simulink model "analog_ext2"  (Simulink 7.6)
settings: Solver=FixedStepDiscrete  StartTime=0.0  StopTime=10000  FixedStep=1  RelTol=1e-3
libraries: simulink x8
settings Model: Creator=jordan  LastModifiedBy=jordan
settings DataIOCC: LimitDataPoints=off  SaveOutput=off  SignalLogging=off  DSMLogging=off  SaveTime=off
settings OptimizationCC: BlockReduction=off  ConditionallyExecuteInputs=off

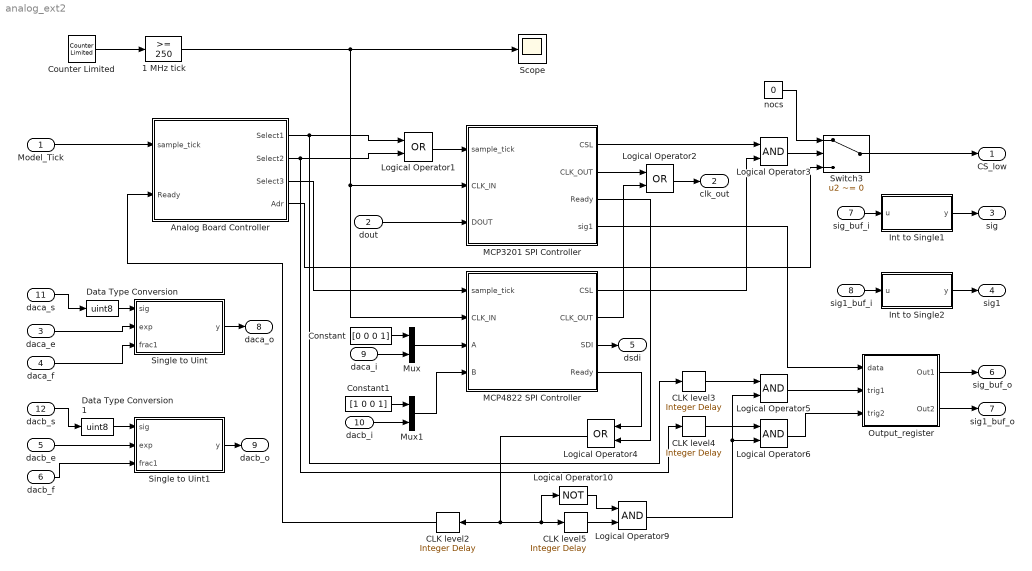
== system analog_ext2 ==
  Model_Tick : Inport  OutDataTypeStr=boolean
  dout : Inport  Port=2  OutDataTypeStr=boolean
  daca_e : Inport  Port=3  OutDataTypeStr=uint8
  daca_f : Inport  Port=4  OutDataTypeStr=fixdt(0,24,0)
  dacb_e : Inport  Port=5  OutDataTypeStr=uint8
  dacb_f : Inport  Port=6  OutDataTypeStr=fixdt(0,24,0)
  sig_buf_i : Inport  Port=7  OutDataTypeStr=fixdt(0,12,0)
  sig1_buf_i : Inport  Port=8  OutDataTypeStr=fixdt(0,12,0)
  daca_i : Inport  Port=9  OutDataTypeStr=boolean  PortDimensions=12
  dacb_i : Inport  Port=10  OutDataTypeStr=boolean  PortDimensions=12
  daca_s : Inport  Port=11  OutDataTypeStr=boolean
  dacb_s : Inport  Port=12  OutDataTypeStr=boolean
  1 MHz tick : simulink/Logic and Bit Operations/Compare To Constant  SystemSampleTime=-1  relop=>=  const=250  LogicOutDataTypeMode=boolean
  Analog Board Controller : Stateflow chart  TreatAsAtomicUnit=on
  CLK level{2..5} (4 alike) : simulink/Discrete/Integer Delay  NumDelays=1  vinit=0.0  samptime=-1
  Constant : Constant  Value=[0 0 0 1]  OutDataTypeStr=boolean
  Constant1 : Constant  Value=[1 0 0 1]  OutDataTypeStr=boolean
  Counter Limited : simulink/Sources/Counter Limited  SystemSampleTime=-1  uplimit=500  tsamp=-1
  Data Type Conversion : DataTypeConversion  OutDataTypeStr=uint8
  Data Type Conversion1 : DataTypeConversion  OutDataTypeStr=uint8
  Int to Single1 : Stateflow chart  TreatAsAtomicUnit=on
  Int to Single2 : Stateflow chart  TreatAsAtomicUnit=on
  Logical Operator1 : Logic  Operator=OR  AllPortsSameDT=off  OutDataTypeStr=boolean
  Logical Operator10 : Logic  Operator=NOT  AllPortsSameDT=off  OutDataTypeStr=boolean
  Logical Operator2 : Logic  Operator=OR  AllPortsSameDT=off  OutDataTypeStr=boolean
  Logical Operator{3,5..6,9} (4 alike) : Logic  AllPortsSameDT=off  OutDataTypeStr=boolean
  Logical Operator4 : Logic  Operator=OR  AllPortsSameDT=off  OutDataTypeStr=boolean
  MCP3201 SPI Controller : Stateflow chart  TreatAsAtomicUnit=on
  MCP4822 SPI Controller : Stateflow chart  TreatAsAtomicUnit=on
  Mux : Mux  Inputs=2
  Mux1 : Mux  Inputs=2
  Output_register : Subsystem
  Scope : Scope
  Single to Uint : Stateflow chart  TreatAsAtomicUnit=on
  Single to Uint1 : Stateflow chart  TreatAsAtomicUnit=on
  Switch3 : Switch  Criteria=u2 ~= 0
  nocs : Constant  Value=0  OutDataTypeStr=fixdt(0,3,0)
  CS_low : Outport  OutDataTypeStr=fixdt(0,3,0)
  clk_out : Outport  Port=2  OutDataTypeStr=boolean
  sig : Outport  Port=3  OutDataTypeStr=uint32  PortDimensions=1
  sig1 : Outport  Port=4  OutDataTypeStr=uint32  PortDimensions=1
  dsdi : Outport  Port=5  OutDataTypeStr=boolean
  sig_buf_o : Outport  Port=6  OutDataTypeStr=boolean  PortDimensions=12
  sig1_buf_o : Outport  Port=7  OutDataTypeStr=boolean  PortDimensions=12
  daca_o : Outport  Port=8  OutDataTypeStr=fixdt(0,12,0)
  dacb_o : Outport  Port=9  OutDataTypeStr=fixdt(0,12,0)
  wires:
  Counter Limited/1 -> 1 MHz tick/1
  1 MHz tick/1 -> MCP4822 SPI Controller/2(CLK_IN), MCP3201 SPI Controller/2(CLK_IN), Scope/1
  dout/1 -> MCP3201 SPI Controller/3(DOUT)
  Constant/1 -> Mux/1
  Constant1/1 -> Mux1/1
  Output_register/1(Out1) -> sig_buf_o/1
  Output_register/2(Out2) -> sig1_buf_o/1
  Int to Single1/1(y) -> sig/1
  Int to Single2/1(y) -> sig1/1
  Single to Uint/1(y) -> daca_o/1
  Single to Uint1/1(y) -> dacb_o/1
  daca_s/1 -> Data Type Conversion/1
  daca_e/1 -> Single to Uint/2(exp)
  daca_f/1 -> Single to Uint/3(frac1)
  dacb_e/1 -> Single to Uint1/2(exp)
  dacb_f/1 -> Single to Uint1/3(frac1)
  sig_buf_i/1 -> Int to Single1/1(u)
  sig1_buf_i/1 -> Int to Single2/1(u)
  daca_i/1 -> Mux/2
  dacb_i/1 -> Mux1/2
  dacb_s/1 -> Data Type Conversion1/1
  Data Type Conversion/1 -> Single to Uint/1(sig)
  Data Type Conversion1/1 -> Single to Uint1/1(sig)
  Mux/1 -> MCP4822 SPI Controller/3(A)
  Mux1/1 -> MCP4822 SPI Controller/4(B)
  Analog Board Controller/1(Select1) -> Logical Operator1/1, CLK level3/1
  Analog Board Controller/2(Select2) -> Logical Operator1/2, CLK level4/1
  Logical Operator1/1 -> MCP3201 SPI Controller/1(sample_tick)
  Analog Board Controller/3(Select3) -> MCP4822 SPI Controller/1(sample_tick)
  Model_Tick/1 -> Analog Board Controller/1(sample_tick)
  MCP3201 SPI Controller/2(CLK_OUT) -> Logical Operator2/1
  Logical Operator2/1 -> clk_out/1
  MCP4822 SPI Controller/2(CLK_OUT) -> Logical Operator2/2
  MCP4822 SPI Controller/3(SDI) -> dsdi/1
  MCP3201 SPI Controller/1(CSL) -> Logical Operator3/1
  MCP4822 SPI Controller/1(CSL) -> Logical Operator3/2
  Logical Operator3/1 -> Switch3/2
  Analog Board Controller/4(Adr) -> Switch3/3
  nocs/1 -> Switch3/1
  Switch3/1 -> CS_low/1
  MCP3201 SPI Controller/3(Ready) -> Logical Operator4/2
  MCP4822 SPI Controller/4(Ready) -> Logical Operator4/1
  Logical Operator4/1 -> CLK level2/1, CLK level5/1, Logical Operator10/1
  CLK level2/1 -> Analog Board Controller/2(Ready)
  Logical Operator5/1 -> Output_register/2(trig1)
  Logical Operator6/1 -> Output_register/3(trig2)
  CLK level5/1 -> Logical Operator9/2
  Logical Operator10/1 -> Logical Operator9/1
  Logical Operator9/1 -> Logical Operator5/2, Logical Operator6/2
  CLK level3/1 -> Logical Operator5/1
  CLK level4/1 -> Logical Operator6/1
  MCP3201 SPI Controller/4(sig1) -> Output_register/1(data)

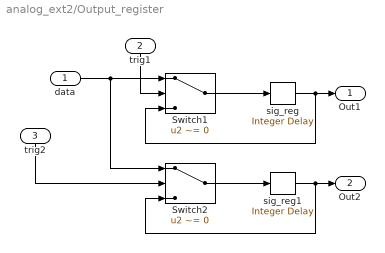
== system analog_ext2/Output_register ==
  data : Inport
  trig1 : Inport  Port=2
  trig2 : Inport  Port=3
  Switch1 : Switch  Criteria=u2 ~= 0
  Switch2 : Switch  Criteria=u2 ~= 0
  sig_reg : simulink/Discrete/Integer Delay  NumDelays=1  vinit=0.0  samptime=-1
  sig_reg1 : simulink/Discrete/Integer Delay  NumDelays=1  vinit=0.0  samptime=-1
  Out1 : Outport
  Out2 : Outport  Port=2
  wires:
  Switch1/1 -> sig_reg/1
  sig_reg/1 -> Switch1/3, Out1/1
  Switch2/1 -> sig_reg1/1
  sig_reg1/1 -> Switch2/3, Out2/1
  trig1/1 -> Switch1/2
  data/1 -> Switch1/1, Switch2/1
  trig2/1 -> Switch2/2

== stateflow chart MCP4822 SPI Controller ==
  settings: executeAtInitialization=1  initializeOutput=1
  state Wait_Request
  state Wait_CLK
  state Wait_CLK_0
  state DAC_A_Send
  state LatchData
  state Buf_state
  state Buf_state1
  state DAC_A_Send1
  state Wait_CLK1
  state Buf_state2
  state Buf_state4
  (default) -> Wait_Request : {CSL=1;
      | CLK_OUT=0;
      | SDI=0;
      | Ready=0;}
  Wait_Request -> Wait_CLK_0 : [sample_tick]{Ready=1;}
  Wait_CLK_0 -> DAC_A_Send : [CLK_IN==0]{
      | CSL=0;
      | CLK_OUT=0;
      | ind=0;
      | SDI=A[0];}
  (junction 14) -> DAC_A_Send
  DAC_A_Send -> Wait_CLK : [CLK_IN]{
      | CLK_OUT=1;
      | ind++;}
  LatchData -> Buf_state2 : [CLK_IN]
  Buf_state2 -> Buf_state4 : [CLK_IN==0]{Ready=0;}
  Wait_CLK -> (junction 15) : [CLK_IN==0]
  (junction 15) -> (junction 14) [order 2] : {CLK_OUT=0;
      | SDI=A[ind];}
  (junction 15) -> Buf_state [order 1] : [ind==16]{CLK_OUT=0;CSL=1;}
  Buf_state -> Buf_state1 : [CLK_IN]
  DAC_A_Send1 -> Wait_CLK1 : [CLK_IN]{
      | CLK_OUT=1;
      | ind++;}
  Wait_CLK1 -> (junction 16) : [CLK_IN==0]
  (junction 16) -> (junction 17) [order 2] : {CLK_OUT=0;
      | SDI=B[ind];}
  (junction 17) -> DAC_A_Send1
  Buf_state1 -> DAC_A_Send1 : [CLK_IN==0]{
      | CSL=0;
      | ind=0;
      | SDI=B[0];}
  (junction 16) -> LatchData [order 1] : [ind==16]{CLK_OUT=0;CSL=1;}
  Buf_state4 -> Wait_Request
  data: sample_tick input boolean; CSL output boolean; CLK_OUT output boolean; CLK_IN input boolean; A input boolean size=16; ind local fixdt(0,5,0); B input boolean size=16; SDI output boolean; Ready output boolean

== stateflow chart MCP3201 SPI Controller ==
  settings: executeAtInitialization=1  initializeOutput=1
  state Wait_Request
    du: CSL=1; CLK_OUT=0; Ready=0; sig1=sig;
  state Get_Sample
    du: CSL=0;CLK_OUT=0;
  state Wait_CLK_0
    du: Ready=1; sig=0;
  state Get_Sample1
    du: CLK_OUT=1;
  state Get_Sample2
    du: CLK_OUT=0;
  state Get_Sample3
    du: CLK_OUT=1;
  state Receive_Data
    du: CLK_OUT=0;
  state Receive_Data1
    du: CLK_OUT=1;
  state Receive_Data2
    du: CLK_OUT=1;
  state Get_Sample4
    du: CLK_OUT=0;
  state Get_Sample5
    du: CLK_OUT=1;
  state Receive_Data3
    du: CLK_OUT=0; CSL=1; sig1=sig;
  state Receive_Data4
    du: Ready=0; CSL=1; CLK_OUT=0; sig1=sig;
  (default) -> Wait_Request
  Wait_Request -> Wait_CLK_0 : [sample_tick]
  Wait_CLK_0 -> Get_Sample : [CLK_IN==0]
  Get_Sample -> Get_Sample1 : [CLK_IN]
  Get_Sample1 -> Get_Sample2 : [CLK_IN==0]
  Get_Sample2 -> Get_Sample3 : [CLK_IN]
  Get_Sample3 -> Get_Sample4 : [CLK_IN==0]
  Receive_Data -> (junction 60) : [CLK_IN]{
      | sig[ind]=DOUT;}
  (junction 60) -> (junction 61)
  (junction 61) -> Receive_Data1 [order 2]
  Receive_Data1 -> Receive_Data : [CLK_IN==0]{ind++;}
  (junction 61) -> Receive_Data2 [order 1] : [ind==11]
  Receive_Data2 -> (junction 62) : [CLK_IN==0]
  (junction 62) -> Receive_Data3
  Get_Sample4 -> Get_Sample5 : [CLK_IN]
  Get_Sample5 -> (junction 63) : [CLK_IN==0]{ind=0;}
  (junction 63) -> Receive_Data
  Receive_Data3 -> Receive_Data4 : [CLK_IN]
  Receive_Data4 -> Wait_Request : [CLK_IN==0]
  data: sample_tick input boolean; CSL output boolean; CLK_OUT output boolean; CLK_IN input boolean; DOUT input boolean; sig local boolean size=12; ind local fixdt(0,4,0); Ready output boolean; sig1 output boolean size=12

== matlab function Int to Single1 ==
  data: u input fixdt(0,12,0); y output uint32
function y = fcn(u)
%#eml

sig=uint8(0);
exp=uint8(0);
frac=fi(0,0,23,0);

%Transform two's complement integer into unnormalized
%single number
buf=fi(0,0,12,0);
sig=uint8(0);
buf=u;
frac1=fi(buf,0,23,0);

%Normalize floating-point number
buf1=fi(frac1,0,24,0);
p=fi(0,0,5,0);
mask=fi(2^22,0,24,0);
for ind=1:23
    c=bitand(buf1,mask);
    if (c==0)
        buf1=bitshift(buf1,1);
        p=fi(p+1,0,5,0);
    end
end
p=fi(p+1,0,5,0);
buf1=bitshift(fi(frac1,0,24,0),uint8(p));
mask1=fi(2^23-1,0,24,0);
buf1=bitand(buf1,mask1);
frac=fi(buf1,0,23,0);
exp=uint8(127+(22-p));

%Compose floating-point number
z=uint32(0);
if sig
    z=uint32(bitshift(uint32(1),31));
end
buf2=uint32(bitshift(uint32(exp),23));
z=bitor(z,buf2);
z=bitor(z,uint32(frac));
y=z;

== matlab function Int to Single2 ==
  data: u input fixdt(0,12,0); y output uint32
function y = fcn(u)
%#eml

sig=uint8(0);
exp=uint8(0);
frac=fi(0,0,23,0);

%Transform two's complement integer into unnormalized
%single number
buf=fi(0,0,12,0);
sig=uint8(0);
buf=u;
frac1=fi(buf,0,23,0);

%Normalize floating-point number
buf1=fi(frac1,0,24,0);
p=fi(0,0,5,0);
mask=fi(2^22,0,24,0);
for ind=1:23
    c=bitand(buf1,mask);
    if (c==0)
        buf1=bitshift(buf1,1);
        p=fi(p+1,0,5,0);
    end
end
p=fi(p+1,0,5,0);
buf1=bitshift(fi(frac1,0,24,0),uint8(p));
mask1=fi(2^23-1,0,24,0);
buf1=bitand(buf1,mask1);
frac=fi(buf1,0,23,0);
exp=uint8(127+(22-p));

%Compose floating-point number
z=uint32(0);
if sig
    z=uint32(bitshift(uint32(1),31));
end
buf2=uint32(bitshift(uint32(exp),23));
z=bitor(z,buf2);
z=bitor(z,uint32(frac));
y=z;

== matlab function Single to Uint ==
  data: sig input uint8; y output fixdt(0,12,0); exp input uint8; frac1 input fixdt(0,24,0)
function y = fcn(sig, exp, frac1)
%#eml

y=fi(0,0,12,0);
z=int16(0);
if (sig==0)
    if (exp>=127)
        buf=uint32(frac1);
        z=int16(exp)-150;
        y=fi(bitshift(buf,z),0,12,0); %-23+(exp-127)
    end
end

== matlab function Single to Uint1 ==
  data: sig input uint8; y output fixdt(0,12,0); exp input uint8; frac1 input fixdt(0,24,0)
function y = fcn(sig, exp, frac1)
%#eml

y=fi(0,0,12,0);
z=int16(0);
if (sig==0)
    if (exp>=127)
        buf=uint32(frac1);
        z=int16(exp)-150;
        y=fi(bitshift(buf,z),0,12,0); %-23+(exp-127)
    end
end

== stateflow chart Analog Board Controller ==
  settings: executeAtInitialization=1  initializeOutput=1
  state Wait_Request
  state Wait6
  state ADC1
  state Wait4
  state Wait2
  state Wait
  state DAC12
  state ADC2
  state Wait3
  (default) -> Wait_Request : {Select1=0;Select2=0;Select3=0;Adr=0;}
  Wait_Request -> ADC1 : [sample_tick]{
      | Select1=1;
      | Select2=0;
      | Select3=0;
      | Adr=6;}
  Wait6 -> Wait_Request : [Ready==0]{
      | Select1=0;
      | Select2=0;
      | Select3=0;
      | Adr=0;}
  ADC2 -> Wait4 : [Ready]
  Wait -> Wait2 : [Ready==0]
  ADC1 -> Wait : [Ready]
  DAC12 -> Wait6 : [Ready]
  Wait2 -> ADC2 : {Select1=0;
      | Select2=1;
      | Select3=0;
      | Adr=5;}
  Wait4 -> Wait3 : [Ready==0]
  Wait3 -> DAC12 : {Select1=0;
      | Select2=0;
      | Select3=1;
      | Adr=7;}
  data: sample_tick input boolean; Select1 output boolean; Ready input boolean; Select2 output boolean; Select3 output boolean; Adr output fixdt(0,3,0)
